simulink model "Aim_23__Monocopter_Testing"  (R2023b)
settings: Solver=ode23t  StartTime=0.0  StopTime=10  MaxStep=1e-3  RelTol=1e-3  AbsTol=1e-3
values from neighbouring files (symbols this model uses):
  air_rho = 1.225    [Aim_23_inherited_params.mat]
  battery_capacity = 22.8    [Aim_23_inherited_params.mat]
  CDO = 10.25    [Aim_23_inherited_params.mat]
  drag_linear = 0.002    [Aim_23_inherited_params.mat]
  drag_quad = 0.005    [Aim_23_inherited_params.mat]
  filtD_motor = 100    [Aim_23_inherited_params.mat]
  filtSpd_motor = 0.001    [Aim_23_inherited_params.mat]
  flap_radius = 0.05312    [Aim_23_inherited_params.mat]
  flap_surface_area = 0.025    [Aim_23_inherited_params.mat]
  kd_motor = 0    [Aim_23_inherited_params.mat]
  ki_motor = 0.00045    [Aim_23_inherited_params.mat]
  klinear = 0.03    [Aim_23_inherited_params.mat]
  kquad = 0.025    [Aim_23_inherited_params.mat]
  limit_motor = 0.25    [Aim_23_inherited_params.mat]
  monoco_mass = 160    [Aim_23_inherited_params.mat]
  monoco_prop =     [Aim_23_inherited_params.mat]
  monoco_radius = 0.61    [Aim_23_inherited_params.mat]
  monoco_wing =     [Aim_23_inherited_params.mat]
  monoco_wing_area = 0.239    [Aim_23_inherited_params.mat]
  waypoints = [-2 -2 0.14 -2 -2 6 0 0 6 2 0 6 ... (15 elements, 3x5)]    [Aim_23_inherited_params.mat]
undefined symbols (not defined in the file or in its folder): X, Y, Z
libraries: sm_lib x97, nesl_utility x38, slpidlib x18, fl_lib x12, sdl_lib x3, simulink x2, simulink_extras x1, batteryecm_lib x1, ee_lib x1
(part 5 of 7)

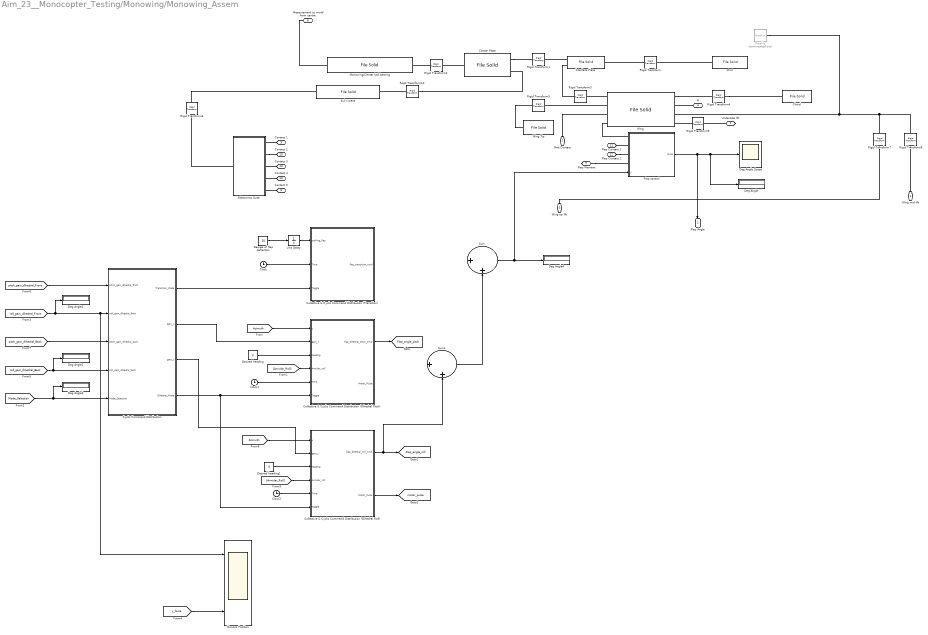
== system Aim_23__Monocopter_Testing/Monowing/Monowing_Assem ==
  " strut" : sm_lib/Body Elements/File Solid  ExtGeomFileName=C:\Users\emman\Monocopter_Frame\DmMc_3mmCF_Strut.STEP  UnitType=FromFile  ExtGeomFileUnits=m  StepReaderType=HEX  ExportConvexHullGeometry=off  InertiaType=CalculateFromGeometry  Mass=5.63  MassUnits=g  CenterOfMass=[0 0 0]  CenterOfMassUnits=m  MomentsOfInertia=[1 1 1]  MomentsOfInertiaUnits=kg*m^2  ProductsOfInertia=[0 0 0]  ProductsOfInertiaUnits=kg*m^2  BasedOnType=Mass  Density=1000  DensityUnits=kg/m^3  DoExposeReferenceFrame=off  SerializedFrames=<Frames><Frame><Id>Frame1</Id><Value><Name>interface</Name><Origin><Source>GeometricFeature</Source><FeatureName>planar surface 6</FeatureName></Origin><PrimaryAxis><DefinedDirection>+Z</DefinedDirection><Source>ReferenceFrame</Source><SourceDirection>+Z</SourceDirection><FeatureName></FeatureName></PrimaryAxis><SecondaryAxis><DefinedDirection>+X</DefinedDirection><Source>ReferenceFrame</Source><SourceDirection>+X</SourceDirection><FeatureName></FeatureName></SecondaryAxis></Value></Frame></Frames>  GraphicType=FromGeometry  MarkerShape=Sphere  MarkerSize=10  GraphicVisPropType=SimpleVisualProperties  GraphicDiffuseColor=[0.5 0.5 0.5]  GraphicSpecularColor=[0.5 0.5 0.5 1.0]  GraphicAmbientColor=[0.15 0.15 0.15 1.0]  GraphicEmissiveColor=[0.0 0.0 0.0 1.0]  GraphicShininess=75  GraphicOpacity=1.0
  Center Plate : sm_lib/Body Elements/File Solid  ExtGeomFileName=C:\Users\emman\Monocopter_Frame\DmMc_center_plate.STEP  UnitType=FromFile  ExtGeomFileUnits=m  StepReaderType=HEX  ExportConvexHullGeometry=off  InertiaType=CalculateFromGeometry  Mass=16.60  MassUnits=g  CenterOfMass=[0 0 0]  CenterOfMassUnits=m  MomentsOfInertia=[1 1 1]  MomentsOfInertiaUnits=kg*m^2  ProductsOfInertia=[0 0 0]  ProductsOfInertiaUnits=kg*m^2  BasedOnType=Mass  Density=1000  DensityUnits=kg/m^3  DoExposeReferenceFrame=on  SerializedFrames=<Frames><Frame><Id>Frame2</Id><Value><Name>interface</Name><Origin><Source>CenterOfMassFrame</Source><FeatureName></FeatureName></Origin><PrimaryAxis><DefinedDirection>+Z</DefinedDirection><Source>ReferenceFrame</Source><SourceDirection>+Z</SourceDirection><FeatureName></FeatureName></PrimaryAxis><SecondaryAxis><DefinedDirection>+X</DefinedDirection><Source>ReferenceFrame</Source><SourceDirection>+X</SourceDirection><FeatureName></FeatureName></SecondaryAxis></Value></Frame><Frame><Id>Frame3</Id><Value><Name>kukri</Name><Origin><Source>CenterOfMassFrame</Source><FeatureName></FeatureName></Origin><PrimaryAxis><DefinedDirection>+Z</DefinedDirection><Source>ReferenceFrame</Source><SourceDirection>+Z</SourceDirection><FeatureName></FeatureName></PrimaryAxis><SecondaryAxis><DefinedDirection>+X</DefinedDirection><Source>ReferenceFrame</Source><SourceDirection>+X</SourceDirection><FeatureName></FeatureName></SecondaryAxis></Value></Frame></Frames>  GraphicType=FromGeometry  MarkerShape=Sphere  MarkerSize=10  GraphicVisPropType=SimpleVisualProperties  GraphicDiffuseColor=[0.5 0.5 0.5]  GraphicSpecularColor=[0.5 0.5 0.5 1.0]  GraphicAmbientColor=[0.15 0.15 0.15 1.0]  GraphicEmissiveColor=[0.0 0.0 0.0 1.0]  GraphicShininess=75  GraphicOpacity=1.0
  Chord : sm_lib/Body Elements/File Solid  ExtGeomFileName=C:\Users\emman\Monocopter_Frame\servo_kukri.STEP  UnitType=FromFile  ExtGeomFileUnits=m  StepReaderType=HEX  ExportConvexHullGeometry=off  InertiaType=CalculateFromGeometry  Mass=8.42  MassUnits=g  CenterOfMass=[0 0 0]  CenterOfMassUnits=m  MomentsOfInertia=[1 1 1]  MomentsOfInertiaUnits=kg*m^2  ProductsOfInertia=[0 0 0]  ProductsOfInertiaUnits=kg*m^2  BasedOnType=Mass  Density=1000  DensityUnits=kg/m^3  DoExposeReferenceFrame=off  SerializedFrames=<Frames><Frame><Id>Frame1</Id><Value><Name>wing</Name><Origin><Source>GeometricFeature</Source><FeatureName>cylindrical surface 54</FeatureName></Origin><PrimaryAxis><DefinedDirection>+Z</DefinedDirection><Source>ReferenceFrame</Source><SourceDirection>+Z</SourceDirection><FeatureName></FeatureName></PrimaryAxis><SecondaryAxis><DefinedDirection>+X</DefinedDirection><Source>ReferenceFrame</Source><SourceDirection>+X</SourceDirection><FeatureName></FeatureName></SecondaryAxis></Value></Frame></Frames>  GraphicType=FromGeometry  MarkerShape=Sphere  MarkerSize=10  GraphicVisPropType=SimpleVisualProperties  GraphicDiffuseColor=[0.5 0.5 0.5]  GraphicSpecularColor=[0.5 0.5 0.5 1.0]  GraphicAmbientColor=[0.15 0.15 0.15 1.0]  GraphicEmissiveColor=[0.0 0.0 0.0 1.0]  GraphicShininess=75  GraphicOpacity=1.0
  Clock : Clock
  Clock1 : Clock
  Clock2 : Clock
  Collective & Cyclic Command Distribution (Dihedral Pitch) : MATLAB Function  TreatAsAtomicUnit=on
  Collective & Cyclic Command Distribution (Dihedral Roll) : MATLAB Function  TreatAsAtomicUnit=on
  Collective & Cyclic Command Distribution (Transition) : MATLAB Function  TreatAsAtomicUnit=on
  Cyclic Command Distribution : MATLAB Function  TreatAsAtomicUnit=on
  Deg Angle{,1..4} (5 alike) : Display
  Deg Angle Scope : Scope
  Degree of flap deflection : Constant  Value=20
  Desired heading : Constant  Value=0
  Desired heading1 : Constant  Value=0
  Electronics Suite : Subsystem
  Flap control : Subsystem
      settings: PortSchema="{\"entries\":[{\"content\":{\"sides\":[{\"content\":{\"connectorIds\":[\"LConn1\",\"LConn2\",\"LConn3\",\"LConn4\",\"In1\"]},\"type\":\"ConnectorPlacement.EquallySpacedRectSide\",\"uuid\":\"1c7c147e-07d6-4292-8f44-26cc109a5078\"},{\"content\":{\"connectorIds\":[\"Out1\"],\"side\":\"RIGHT\"},\"type\":\"ConnectorPlacement.EquallySpacedRectSide\",\"uuid\":\"69a37138-836f-4c0d-80a7-fdf15f5e4c6b\"},{\"content\":{\"connectorIds\":[],\"side\":\"TOP\"},\"type\":\"ConnectorPlacement.EquallySpacedRectSide\",\"uuid\":\"e764985a-8534-4fec-879a-c3123f61d064\"}]},\"type\":\"ConnectorPlacement.EquallySpacedConnector\",\"uuid\":\"d5bc741b-53d2-45d8-8f6d-90823476833a\"}],\"packageUris\":[\"http://schema.mathworks.com/mf0/Connector/R2020b\"],\"version\":\"1.0\"}"
  Graphic : sm_lib/Body Elements/Graphic  Commented=on  GraphicType=Marker  MarkerShape=Cube  MarkerSize=10  GraphicVisPropType=AdvancedVisualProperties  GraphicDiffuseColor=[0.5 0.5 0.5]  GraphicSpecularColor=[0.5 0.5 0.5 1.0]  GraphicAmbientColor=[0.15 0.15 0.15 1.0]  GraphicEmissiveColor=[0.0 0.0 0.0 1.0]  GraphicShininess=75  GraphicOpacity=1.0
  Interface Plate : sm_lib/Body Elements/File Solid  ExtGeomFileName=C:\Users\emman\Monocopter_Frame\new_mid.STEP  UnitType=FromFile  ExtGeomFileUnits=m  StepReaderType=HEX  ExportConvexHullGeometry=off  InertiaType=CalculateFromGeometry  Mass=9.07  MassUnits=g  CenterOfMass=[0 0 0]  CenterOfMassUnits=m  MomentsOfInertia=[1 1 1]  MomentsOfInertiaUnits=kg*m^2  ProductsOfInertia=[0 0 0]  ProductsOfInertiaUnits=kg*m^2  BasedOnType=Mass  Density=1000  DensityUnits=kg/m^3  DoExposeReferenceFrame=off  SerializedFrames=<Frames><Frame><Id>Frame1</Id><Value><Name>interface</Name><Origin><Source>CenterOfMassFrame</Source><FeatureName></FeatureName></Origin><PrimaryAxis><DefinedDirection>+Z</DefinedDirection><Source>ReferenceFrame</Source><SourceDirection>+Z</SourceDirection><FeatureName></FeatureName></PrimaryAxis><SecondaryAxis><DefinedDirection>+X</DefinedDirection><Source>ReferenceFrame</Source><SourceDirection>+X</SourceDirection><FeatureName></FeatureName></SecondaryAxis></Value></Frame><Frame><Id>Frame2</Id><Value><Name>strut</Name><Origin><Source>GeometricFeature</Source><FeatureName>planar surface 30</FeatureName></Origin><PrimaryAxis><DefinedDirection>+Z</DefinedDirection><Source>ReferenceFrame</Source><SourceDirection>+Z</SourceDirection><FeatureName></FeatureName></PrimaryAxis><SecondaryAxis><DefinedDirection>+X</DefinedDirection><Source>ReferenceFrame</Source><SourceDirection>+X</SourceDirection><FeatureName></FeatureName></SecondaryAxis></Value></Frame><Frame><Id>Frame3</Id><Value><Name>wing</Name><Origin><Source>GeometricFeature</Source><FeatureName>planar surface 23</FeatureName></Origin><PrimaryAxis><DefinedDirection>+Z</DefinedDirection><Source>ReferenceFrame</Source><SourceDirection>+Z</SourceDirection><FeatureName></FeatureName></PrimaryAxis><SecondaryAxis><DefinedDirection>+X</DefinedDirection><Source>ReferenceFrame</Source><SourceDirection>+X</SourceDirection><FeatureName></FeatureName></SecondaryAxis></Value></Frame></Frames>  GraphicType=FromGeometry  MarkerShape=Sphere  MarkerSize=10  GraphicVisPropType=SimpleVisualProperties  GraphicDiffuseColor=[0.5 0.5 0.5]  GraphicSpecularColor=[0.5 0.5 0.5 1.0]  GraphicAmbientColor=[0.15 0.15 0.15 1.0]  GraphicEmissiveColor=[0.0 0.0 0.0 1.0]  GraphicShininess=75  GraphicOpacity=1.0
  Kukri piece : sm_lib/Body Elements/File Solid  ExtGeomFileName=C:\Users\emman\Monocopter_Frame\kukri_mid.STEP  UnitType=FromFile  ExtGeomFileUnits=m  StepReaderType=HEX  ExportConvexHullGeometry=off  InertiaType=CalculateFromGeometry  Mass=17.68  MassUnits=g  CenterOfMass=[0 0 0]  CenterOfMassUnits=m  MomentsOfInertia=[1 1 1]  MomentsOfInertiaUnits=kg*m^2  ProductsOfInertia=[0 0 0]  ProductsOfInertiaUnits=kg*m^2  BasedOnType=Mass  Density=1000  DensityUnits=kg/m^3  DoExposeReferenceFrame=off  SerializedFrames=<Frames><Frame><Id>Frame1</Id><Value><Name>Electronics</Name><Origin><Source>GeometricFeature</Source><FeatureName>planar surface 7</FeatureName></Origin><PrimaryAxis><DefinedDirection>+Z</DefinedDirection><Source>ReferenceFrame</Source><SourceDirection>+Z</SourceDirection><FeatureName></FeatureName></PrimaryAxis><SecondaryAxis><DefinedDirection>+X</DefinedDirection><Source>ReferenceFrame</Source><SourceDirection>+X</SourceDirection><FeatureName></FeatureName></SecondaryAxis></Value></Frame><Frame><Id>Frame2</Id><Value><Name>Center_plate</Name><Origin><Source>GeometricFeature</Source><FeatureName>planar surface 11</FeatureName></Origin><PrimaryAxis><DefinedDirection>+Z</DefinedDirection><Source>ReferenceFrame</Source><SourceDirection>+Z</SourceDirection><FeatureName></FeatureName></PrimaryAxis><SecondaryAxis><DefinedDirection>+X</DefinedDirection><Source>ReferenceFrame</Source><SourceDirection>+X</SourceDirection><FeatureName></FeatureName></SecondaryAxis></Value></Frame></Frames>  GraphicType=FromGeometry  MarkerShape=Sphere  MarkerSize=10  GraphicVisPropType=SimpleVisualProperties  GraphicDiffuseColor=[0.5 0.5 0.5]  GraphicSpecularColor=[0.5 0.5 0.5 1.0]  GraphicAmbientColor=[0.15 0.15 0.15 1.0]  GraphicEmissiveColor=[0.0 0.0 0.0 1.0]  GraphicShininess=75  GraphicOpacity=1.0
  Monoco Position : Scope  NumInputPorts=3
  Monowing/Center ball bearing : sm_lib/Body Elements/File Solid  ExtGeomFileName=C:\Users\emman\Monocopter_Frame\DmMc_Ball_Bearing.STEP  UnitType=FromFile  ExtGeomFileUnits=m  StepReaderType=HEX  ExportConvexHullGeometry=off  InertiaType=CalculateFromGeometry  Mass=3.04  MassUnits=g  CenterOfMass=[0 0 0]  CenterOfMassUnits=m  MomentsOfInertia=[0.0001 0.001 0.001]  MomentsOfInertiaUnits=kg*m^2  ProductsOfInertia=[0 0 0]  ProductsOfInertiaUnits=kg*m^2  BasedOnType=Mass  Density=1000  DensityUnits=kg/m^3  DoExposeReferenceFrame=on  SerializedFrames=<Frames><Frame><Id>Frame1</Id><Value><Name>Measurement to world</Name><Origin><Source>ReferenceFrame</Source><FeatureName></FeatureName></Origin><PrimaryAxis><DefinedDirection>+Z</DefinedDirection><Source>ReferenceFrame</Source><SourceDirection>+Z</SourceDirection><FeatureName></FeatureName></PrimaryAxis><SecondaryAxis><DefinedDirection>+X</DefinedDirection><Source>ReferenceFrame</Source><SourceDirection>+X</SourceDirection><FeatureName></FeatureName></SecondaryAxis></Value></Frame></Frames>  GraphicType=FromGeometry  MarkerShape=Sphere  MarkerSize=10  GraphicVisPropType=SimpleVisualProperties  GraphicDiffuseColor=[0.2 0.2 0.2]  GraphicSpecularColor=[0.5 0.5 0.5 1.0]  GraphicAmbientColor=[0.15 0.15 0.15 1.0]  GraphicEmissiveColor=[0.0 0.0 0.0 1.0]  GraphicShininess=75  GraphicOpacity=1.0
  Rigid Transform : sm_lib/Frames and Transforms/Rigid Transform  TranslationMethod=Cartesian  TranslationStandardOffset=0  TranslationStandardOffsetUnits=mm  TranslationStandardAxis=+Z  TranslationCartesianOffset=[0 0 0]  TranslationCartesianOffsetUnits=mm  TranslationROffset=0  TranslationROffsetUnits=m  TranslationZOffset=0  TranslationZOffsetUnits=m  TranslationThetaOffset=0  TranslationThetaOffsetUnits=deg  RotationMethod=RotationSequence  RotationAngleUnits=deg  RotationStandardAxis=+Z  RotationAngle=0.0  RotationArbitraryAxis=[0 0 1]  FollAlignAxisA=+X  BaseAlignAxisA=+Y  FollAlignAxisB=+Y  BaseAlignAxisB=+Z  RotationSequenceAxes=FollowerAxes  RotationSequence=YZX  RotationSequenceAngles=[180 1 -11]  RotationSequenceAnglesUnits=deg  RotationMatrix=[1 0 0; 0 1 0; 0 0 1]  Quaternion=[1 0 0 0]
  Rigid Transform1 : sm_lib/Frames and Transforms/Rigid Transform  TranslationMethod=Cartesian  TranslationStandardOffset=0  TranslationStandardOffsetUnits=mm  TranslationStandardAxis=+Z  TranslationCartesianOffset=[47 -2.5 1.2]  TranslationCartesianOffsetUnits=mm  TranslationROffset=0  TranslationROffsetUnits=m  TranslationZOffset=0  TranslationZOffsetUnits=m  TranslationThetaOffset=0  TranslationThetaOffsetUnits=deg  RotationMethod=RotationSequence  RotationAngleUnits=deg  RotationStandardAxis=+Z  RotationAngle=0.0  RotationArbitraryAxis=[0 0 1]  FollAlignAxisA=+X  BaseAlignAxisA=+Y  FollAlignAxisB=+Y  BaseAlignAxisB=+Z  RotationSequenceAxes=FollowerAxes  RotationSequence=ZXZ  RotationSequenceAngles=[180 0 0]  RotationSequenceAnglesUnits=deg  RotationMatrix=[1 0 0; 0 1 0; 0 0 1]  Quaternion=[1 0 0 0]
  Rigid Transform10 : sm_lib/Frames and Transforms/Rigid Transform  TranslationMethod=Cartesian  TranslationStandardOffset=0  TranslationStandardOffsetUnits=mm  TranslationStandardAxis=+Z  TranslationCartesianOffset=[-27.5 0 0]  TranslationCartesianOffsetUnits=mm  TranslationROffset=0  TranslationROffsetUnits=m  TranslationZOffset=0  TranslationZOffsetUnits=m  TranslationThetaOffset=0  TranslationThetaOffsetUnits=deg  RotationMethod=None  RotationAngleUnits=deg  RotationStandardAxis=+Z  RotationAngle=0.0  RotationArbitraryAxis=[0 0 1]  FollAlignAxisA=+X  BaseAlignAxisA=+Y  FollAlignAxisB=+Y  BaseAlignAxisB=+Z  RotationSequenceAxes=FollowerAxes  RotationSequence=XYX  RotationSequenceAngles=[0 0 0]  RotationSequenceAnglesUnits=deg  RotationMatrix=[1 0 0; 0 1 0; 0 0 1]  Quaternion=[1 0 0 0]
  Rigid Transform2 : sm_lib/Frames and Transforms/Rigid Transform  TranslationMethod=Cartesian  TranslationStandardOffset=0  TranslationStandardOffsetUnits=mm  TranslationStandardAxis=+Z  TranslationCartesianOffset=[0 0 -4]  TranslationCartesianOffsetUnits=mm  TranslationROffset=0  TranslationROffsetUnits=m  TranslationZOffset=0  TranslationZOffsetUnits=m  TranslationThetaOffset=0  TranslationThetaOffsetUnits=deg  RotationMethod=None  RotationAngleUnits=deg  RotationStandardAxis=+Z  RotationAngle=0.0  RotationArbitraryAxis=[0 0 1]  FollAlignAxisA=+X  BaseAlignAxisA=+Y  FollAlignAxisB=+Y  BaseAlignAxisB=+Z  RotationSequenceAxes=FollowerAxes  RotationSequence=XYX  RotationSequenceAngles=[0 0 0]  RotationSequenceAnglesUnits=deg  RotationMatrix=[1 0 0; 0 1 0; 0 0 1]  Quaternion=[1 0 0 0]
  Rigid Transform3 : sm_lib/Frames and Transforms/Rigid Transform  TranslationMethod=Cartesian  TranslationStandardOffset=0  TranslationStandardOffsetUnits=mm  TranslationStandardAxis=+Z  TranslationCartesianOffset=[-186.3 -36.8 7.7]  TranslationCartesianOffsetUnits=mm  TranslationROffset=0  TranslationROffsetUnits=m  TranslationZOffset=0  TranslationZOffsetUnits=m  TranslationThetaOffset=0  TranslationThetaOffsetUnits=deg  RotationMethod=RotationSequence  RotationAngleUnits=deg  RotationStandardAxis=+Z  RotationAngle=0.0  RotationArbitraryAxis=[0 0 1]  FollAlignAxisA=+X  BaseAlignAxisA=+Y  FollAlignAxisB=+Y  BaseAlignAxisB=+Z  RotationSequenceAxes=FollowerAxes  RotationSequence=XYX  RotationSequenceAngles=[-12 0 0]  RotationSequenceAnglesUnits=deg  RotationMatrix=[1 0 0; 0 1 0; 0 0 1]  Quaternion=[1 0 0 0]
  Rigid Transform4 : sm_lib/Frames and Transforms/Rigid Transform  TranslationMethod=Cartesian  TranslationStandardOffset=0  TranslationStandardOffsetUnits=mm  TranslationStandardAxis=+Z  TranslationCartesianOffset=[0.4 5 0.6]  TranslationCartesianOffsetUnits=mm  TranslationROffset=0  TranslationROffsetUnits=m  TranslationZOffset=0  TranslationZOffsetUnits=m  TranslationThetaOffset=0  TranslationThetaOffsetUnits=deg  RotationMethod=RotationSequence  RotationAngleUnits=deg  RotationStandardAxis=+Z  RotationAngle=0.0  RotationArbitraryAxis=[0 0 1]  FollAlignAxisA=+X  BaseAlignAxisA=+Y  FollAlignAxisB=+Y  BaseAlignAxisB=+Z  RotationSequenceAxes=FollowerAxes  RotationSequence=XYX  RotationSequenceAngles=[10 2 0]  RotationSequenceAnglesUnits=deg  RotationMatrix=[1 0 0; 0 1 0; 0 0 1]  Quaternion=[1 0 0 0]
  Rigid Transform5 : sm_lib/Frames and Transforms/Rigid Transform  TranslationMethod=Cartesian  TranslationStandardOffset=0  TranslationStandardOffsetUnits=mm  TranslationStandardAxis=+Z  TranslationCartesianOffset=[6 14.65 3.1]  TranslationCartesianOffsetUnits=mm  TranslationROffset=0  TranslationROffsetUnits=m  TranslationZOffset=0  TranslationZOffsetUnits=m  TranslationThetaOffset=0  TranslationThetaOffsetUnits=deg  RotationMethod=RotationSequence  RotationAngleUnits=deg  RotationStandardAxis=+Z  RotationAngle=0.0  RotationArbitraryAxis=[0 0 1]  FollAlignAxisA=+X  BaseAlignAxisA=+Y  FollAlignAxisB=+Y  BaseAlignAxisB=+Z  RotationSequenceAxes=FollowerAxes  RotationSequence=XYX  RotationSequenceAngles=[12 2 0]  RotationSequenceAnglesUnits=deg  RotationMatrix=[1 0 0; 0 1 0; 0 0 1]  Quaternion=[1 0 0 0]
  Rigid Transform6 : sm_lib/Frames and Transforms/Rigid Transform  TranslationMethod=Cartesian  TranslationStandardOffset=0  TranslationStandardOffsetUnits=mm  TranslationStandardAxis=+Z  TranslationCartesianOffset=[-72.7 -18.05 2.83]  TranslationCartesianOffsetUnits=mm  TranslationROffset=0  TranslationROffsetUnits=m  TranslationZOffset=0  TranslationZOffsetUnits=m  TranslationThetaOffset=0  TranslationThetaOffsetUnits=deg  RotationMethod=RotationSequence  RotationAngleUnits=deg  RotationStandardAxis=+Z  RotationAngle=0.0  RotationArbitraryAxis=[0 0 1]  FollAlignAxisA=+X  BaseAlignAxisA=+Y  FollAlignAxisB=+Y  BaseAlignAxisB=+Z  RotationSequenceAxes=FollowerAxes  RotationSequence=XYZ  RotationSequenceAngles=[180 180.4 15.0]  RotationSequenceAnglesUnits=deg  RotationMatrix=[1 0 0; 0 1 0; 0 0 1]  Quaternion=[1 0 0 0]
  Rigid Transform7 : sm_lib/Frames and Transforms/Rigid Transform  TranslationMethod=Cartesian  TranslationStandardOffset=0  TranslationStandardOffsetUnits=mm  TranslationStandardAxis=+Z  TranslationCartesianOffset=[0 55 80]  TranslationCartesianOffsetUnits=mm  TranslationROffset=0  TranslationROffsetUnits=m  TranslationZOffset=0  TranslationZOffsetUnits=m  TranslationThetaOffset=0  TranslationThetaOffsetUnits=deg  RotationMethod=RotationSequence  RotationAngleUnits=deg  RotationStandardAxis=+Z  RotationAngle=0.0  RotationArbitraryAxis=[0 0 1]  FollAlignAxisA=+X  BaseAlignAxisA=+Y  FollAlignAxisB=+Y  BaseAlignAxisB=+Z  RotationSequenceAxes=FollowerAxes  RotationSequence=XYZ  RotationSequenceAngles=[10 0 0]  RotationSequenceAnglesUnits=deg  RotationMatrix=[1 0 0; 0 1 0; 0 0 1]  Quaternion=[1 0 0 0]
  Rigid Transform8 : sm_lib/Frames and Transforms/Rigid Transform  TranslationMethod=Cartesian  TranslationStandardOffset=0  TranslationStandardOffsetUnits=mm  TranslationStandardAxis=+Z  TranslationCartesianOffset=[0 60 15]  TranslationCartesianOffsetUnits=mm  TranslationROffset=0  TranslationROffsetUnits=m  TranslationZOffset=0  TranslationZOffsetUnits=m  TranslationThetaOffset=0  TranslationThetaOffsetUnits=deg  RotationMethod=None  RotationAngleUnits=deg  RotationStandardAxis=+Z  RotationAngle=0.0  RotationArbitraryAxis=[0 0 1]  FollAlignAxisA=+X  BaseAlignAxisA=+Y  FollAlignAxisB=+Y  BaseAlignAxisB=+Z  RotationSequenceAxes=FollowerAxes  RotationSequence=XYX  RotationSequenceAngles=[0 0 0]  RotationSequenceAnglesUnits=deg  RotationMatrix=[1 0 0; 0 1 0; 0 0 1]  Quaternion=[1 0 0 0]
  Rigid Transform9 : sm_lib/Frames and Transforms/Rigid Transform  TranslationMethod=None  TranslationStandardOffset=0  TranslationStandardOffsetUnits=m  TranslationStandardAxis=+Z  TranslationCartesianOffset=[0 0 0]  TranslationCartesianOffsetUnits=m  TranslationROffset=0  TranslationROffsetUnits=m  TranslationZOffset=0  TranslationZOffsetUnits=m  TranslationThetaOffset=0  TranslationThetaOffsetUnits=deg  RotationMethod=None  RotationAngleUnits=deg  RotationStandardAxis=+Z  RotationAngle=0.0  RotationArbitraryAxis=[0 0 1]  FollAlignAxisA=+X  BaseAlignAxisA=+Y  FollAlignAxisB=+Y  BaseAlignAxisB=+Z  RotationSequenceAxes=FollowerAxes  RotationSequence=XYX  RotationSequenceAngles=[0 0 0]  RotationSequenceAnglesUnits=deg  RotationMatrix=[1 0 0; 0 1 0; 0 0 1]  Quaternion=[1 0 0 0]
  Sum : Sum  Inputs=|++
  Sum1 : Sum  Inputs=|++
  Unit Delay : UnitDelay  SampleTime=7.2  HasFrameUpgradeWarning=on
  Wing : sm_lib/Body Elements/File Solid  ExtGeomFileName=C:\Users\emman\Monocopter_Frame\DmMc_Wing_type7_Flap.STEP  UnitType=FromFile  ExtGeomFileUnits=m  StepReaderType=HEX  ExportConvexHullGeometry=off  InertiaType=CalculateFromGeometry  Mass=1.98  MassUnits=g  CenterOfMass=[0 0 0]  CenterOfMassUnits=m  MomentsOfInertia=[1 1 1]  MomentsOfInertiaUnits=kg*m^2  ProductsOfInertia=[0 0 0]  ProductsOfInertiaUnits=kg*m^2  BasedOnType=Mass  Density=0.016  DensityUnits=g/cm^3  DoExposeReferenceFrame=off  SerializedFrames=<Frames><Frame><Id>Frame1</Id><Value><Name>interface</Name><Origin><Source>CenterOfMassFrame</Source><FeatureName></FeatureName></Origin><PrimaryAxis><DefinedDirection>+Z</DefinedDirection><Source>ReferenceFrame</Source><SourceDirection>+Z</SourceDirection><FeatureName></FeatureName></PrimaryAxis><SecondaryAxis><DefinedDirection>+X</DefinedDirection><Source>ReferenceFrame</Source><SourceDirection>+X</SourceDirection><FeatureName></FeatureName></SecondaryAxis></Value></Frame><Frame><Id>Frame2</Id><Value><Name>chord</Name><Origin><Source>GeometricFeature</Source><FeatureName>planar surface 25</FeatureName></Origin><PrimaryAxis><DefinedDirection>+Z</DefinedDirection><Source>ReferenceFrame</Source><SourceDirection>+Z</SourceDirection><FeatureName></FeatureName></PrimaryAxis><SecondaryAxis><DefinedDirection>+X</DefinedDirection><Source>ReferenceFrame</Source><SourceDirection>+X</SourceDirection><FeatureName></FeatureName></SecondaryAxis></Value></Frame><Frame><Id>Frame3</Id><Value><Name>Wing Tip</Name><Origin><Source>GeometricFeature</Source><FeatureName>general surface 1</FeatureName></Origin><PrimaryAxis><DefinedDirection>+Z</DefinedDirection><Source>ReferenceFrame</Source><SourceDirection>+Z</SourceDirection><FeatureName></FeatureName></PrimaryAxis><SecondaryAxis><DefinedDirection>+X</DefinedDirection><Source>ReferenceFrame</Source><SourceDirection>+X</SourceDirection><FeatureName></FeatureName></SecondaryAxis></Value></Frame><Frame><Id>Frame4</Id><Value><Name>Mount</Name><Origin><Source>ReferenceFrame</Source><FeatureName></FeatureName></Origin><PrimaryAxis><DefinedDirection>+Z</DefinedDirection><Source>ReferenceFrame</Source><SourceDirection>+Z</SourceDirection><FeatureName></FeatureName></PrimaryAxis><SecondaryAxis><DefinedDirection>+X</DefinedDirection><Source>ReferenceFrame</Source><SourceDirection>+X</SourceDirection><FeatureName></FeatureName></SecondaryAxis></Value></Frame><Frame><Id>Frame5</Id><Value><Name>Gnd_Contact</Name><Origin><Source>GeometricFeature</Source><FeatureName>segment 50</FeatureName></Origin><PrimaryAxis><DefinedDirection>+Z</DefinedDirection><Source>ReferenceFrame</Source><SourceDirection>+Z</SourceDirection><FeatureName></FeatureName></PrimaryAxis><SecondaryAxis><DefinedDirection>+X</DefinedDirection><Source>ReferenceFrame</Source><SourceDirection>+X</SourceDirection><FeatureName></FeatureName></SecondaryAxis></Value></Frame><Frame><Id>Frame6</Id><Value><Name>Lift</Name><Origin><Source>CenterOfMassFrame</Source><FeatureName></FeatureName></Origin><PrimaryAxis><DefinedDirection>+Z</DefinedDirection><Source>ReferenceFrame</Source><SourceDirection>+Z</SourceDirection><FeatureName></FeatureName></PrimaryAxis><SecondaryAxis><DefinedDirection>+X</DefinedDirection><Source>ReferenceFrame</Source><SourceDirection>+X</SourceDirection><FeatureName></FeatureName></SecondaryAxis></Value></Frame><Frame><Id>Frame7</Id><Value><Name>Flap</Name><Origin><Source>GeometricFeature</Source><FeatureName>segment 11</FeatureName></Origin><PrimaryAxis><DefinedDirection>+Z</DefinedDirection><Source>GeometricFeature</Source><SourceDirection>+Z</SourceDirection><FeatureName>segment 11</FeatureName></PrimaryAxis><SecondaryAxis><DefinedDirection>+X</DefinedDirection><Source>ReferenceFrame</Source><SourceDirection>+X</SourceDirection><FeatureName></FeatureName></SecondaryAxis></Value></Frame><Frame><Id>Frame8</Id><Value><Name>Lift_underside</Name><Origin><Source>CenterOfMassFrame</Source><FeatureName></FeatureName></Origin><PrimaryAxis><DefinedDirection>-Z</DefinedDirection><Source>ReferenceFrame</Source><SourceDirection>+Z</SourceDirection><FeatureName></FeatureName></PrimaryAxis><SecondaryAxis><DefinedDirection>+X</DefinedDirection><Source>ReferenceFrame</Source><SourceDirection>+X</SourceDirection><FeatureName></FeatureName></SecondaryAxis></Value></Frame></Frames>  GraphicType=FromGeometry  MarkerShape=Sphere  MarkerSize=10  GraphicVisPropType=SimpleVisualProperties  GraphicDiffuseColor=[1.0 1.0 0.2]  GraphicSpecularColor=[0.5 0.5 0.5 1.0]  GraphicAmbientColor=[0.15 0.15 0.15 1.0]  GraphicEmissiveColor=[0.0 0.0 0.0 1.0]  GraphicShininess=75  GraphicOpacity=1.0
  Wing Tip : sm_lib/Body Elements/File Solid  ExtGeomFileName=C:\Users\emman\Monocopter_Frame\DmMc_Wingtip_Rinforce_type6.STEP  UnitType=FromFile  ExtGeomFileUnits=m  StepReaderType=HEX  ExportConvexHullGeometry=off  InertiaType=CalculateFromGeometry  Mass=2.5  MassUnits=g  CenterOfMass=[0 0 0]  CenterOfMassUnits=m  MomentsOfInertia=[1 1 1]  MomentsOfInertiaUnits=kg*m^2  ProductsOfInertia=[0 0 0]  ProductsOfInertiaUnits=kg*m^2  BasedOnType=Mass  Density=1000  DensityUnits=kg/m^3  DoExposeReferenceFrame=off  SerializedFrames=<Frames><Frame><Id>Frame1</Id><Value><Name>Wing</Name><Origin><Source>GeometricFeature</Source><FeatureName>general surface 8</FeatureName></Origin><PrimaryAxis><DefinedDirection>+Z</DefinedDirection><Source>ReferenceFrame</Source><SourceDirection>+Z</SourceDirection><FeatureName></FeatureName></PrimaryAxis><SecondaryAxis><DefinedDirection>+X</DefinedDirection><Source>ReferenceFrame</Source><SourceDirection>+X</SourceDirection><FeatureName></FeatureName></SecondaryAxis></Value></Frame></Frames>  GraphicType=FromGeometry  MarkerShape=Sphere  MarkerSize=10  GraphicVisPropType=SimpleVisualProperties  GraphicDiffuseColor=[0.5 0.5 0.5]  GraphicSpecularColor=[0.5 0.5 0.5 1.0]  GraphicAmbientColor=[0.15 0.15 0.15 1.0]  GraphicEmissiveColor=[0.0 0.0 0.0 1.0]  GraphicShininess=75  GraphicOpacity=1.0
  Wing mid lift : PMIOPort  Side=Left
  Underside lift : PMIOPort  Port=2  Side=Left
  Wing tip lift : PMIOPort  Port=3  Side=Left
  M : PMIOPort  Port=4  Side=Left
  Flap Moment : PMIOPort  Port=5  Side=Left
  Contact 5 : PMIOPort  Port=6  Side=Left
  Gnd Contact : PMIOPort  Port=7  Side=Right
  Measurement to world from centre : PMIOPort  Port=8  Side=Right
  Contact 1 : PMIOPort  Port=9  Side=Right
  Contact 2 : PMIOPort  Port=10  Side=Right
  Flap Contact 1 : PMIOPort  Port=11  Side=Right
  Flap Contact 2 : PMIOPort  Port=12  Side=Right
  Contact 3 : PMIOPort  Port=13  Side=Right
  Contact 4 : PMIOPort  Port=14  Side=Right
  Flap Angle : Outport
  tag scope: Flap_angle_pitch=global, Flap_angle_roll=global, motor_pulse=global
  wires:
  Flap control/1(Out1) -> Flap Angle/1, Deg Angle/1, Deg Angle Scope/1
  Degree of flap deflection/1 -> Unit Delay/1
  Clock/1 -> Collective & Cyclic Command Distribution (Transition)/2(Time)
  Unit Delay/1 -> Collective & Cyclic Command Distribution (Transition)/1(stalling_flap)
  [Annular_Roll] -> Collective & Cyclic Command Distribution (Dihedral Pitch)/4(Annular_roll)
  Desired heading/1 -> Collective & Cyclic Command Distribution (Dihedral Pitch)/3(heading)
  [Azimuth] -> Collective & Cyclic Command Distribution (Dihedral Pitch)/1(u)
  Clock1/1 -> Collective & Cyclic Command Distribution (Dihedral Pitch)/5(Time)
  Cyclic Command Distribution/1(Transition_Mode) -> Collective & Cyclic Command Distribution (Transition)/3(Toggle)
  Cyclic Command Distribution/2(gain_x) -> Collective & Cyclic Command Distribution (Dihedral Pitch)/2(gain_x)
  [Mode_Selection] -> Cyclic Command Distribution/5(Mode_Selection), Deg Angle3/1
  [roll_gain_dihedral_Front] -> Monoco Position/1, Cyclic Command Distribution/2(roll_gain_dihedral_front), Deg Angle1/1
  [roll_gain_dihedral_Back] -> Deg Angle2/1, Cyclic Command Distribution/4(roll_gain_dihedral_back)
  Sum/1 -> Deg Angle4/1, Flap control/1(y)
  Cyclic Command Distribution/4(Dihedral_Mode) -> Collective & Cyclic Command Distribution (Dihedral Roll)/6(Toggle), Collective & Cyclic Command Distribution (Dihedral Pitch)/6(Toggle)
  [y_force] -> Monoco Position/3
  [pitch_gain_dihedral_Front] -> Cyclic Command Distribution/1(pitch_gain_dihedral_front)
  [pitch_gain_dihedral_Back] -> Cyclic Command Distribution/3(pitch_gain_dihedral_back)
  Cyclic Command Distribution/3(gain_y) -> Collective & Cyclic Command Distribution (Dihedral Roll)/2(gain_y)
  [Azimuth] -> Collective & Cyclic Command Distribution (Dihedral Roll)/1(u)
  Desired heading1/1 -> Collective & Cyclic Command Distribution (Dihedral Roll)/3(heading)
  [Annular_Roll] -> Collective & Cyclic Command Distribution (Dihedral Roll)/4(Annular_roll)
  Clock2/1 -> Collective & Cyclic Command Distribution (Dihedral Roll)/5(Time)
  Collective & Cyclic Command Distribution (Dihedral Pitch)/1(flap_dihedral_pitch_cmd) -> [Flap_angle_pitch]
  Collective & Cyclic Command Distribution (Dihedral Roll)/1(flap_dihedral_roll_cmd) -> [Flap_angle_roll], Sum1/2
  Sum1/1 -> Sum/2
  Collective & Cyclic Command Distribution (Dihedral Roll)/2(Motor_Pulse) -> [motor_pulse]
  connections:
  Rigid Transform4/RConn1 -- Chord/LConn1
  Wing/RConn1 -- Rigid Transform4/LConn1
  Rigid Transform/LConn1 -- Interface Plate/RConn1
  Rigid Transform2/LConn1 -- Monowing/Center ball bearing/RConn1
  Interface Plate/LConn1 -- Rigid Transform1/RConn1
  M/RConn1 -- Wing/RConn2
  Wing/LConn1 -- Rigid Transform3/RConn1
  Wing/LConn2 -- Rigid Transform5/LConn1
  Center Plate/RConn1 -- Rigid Transform2/RConn1
  " strut"/LConn1 -- Rigid Transform/RConn1
  Rigid Transform3/LConn1 -- Interface Plate/LConn2
  Rigid Transform5/RConn1 -- Wing Tip/LConn1
  Center Plate/LConn1 -- Rigid Transform1/LConn1
  Wing/LConn3 -- Gnd Contact/RConn1
  Contact 1/RConn1 -- Electronics Suite/RConn1
  Electronics Suite/LConn1 -- Rigid Transform6/RConn1
  Electronics Suite/RConn2 -- Contact 2/RConn1
  Monowing/Center ball bearing/LConn1 -- Measurement to world from centre/RConn1
  Rigid Transform7/RConn1 -- Wing tip lift/RConn1
  Rigid Transform7/LConn1 -- Wing/RConn3 -- Graphic/RConn1 -- Rigid Transform8/LConn1
  Wing mid lift/RConn1 -- Rigid Transform8/RConn1
  Flap control/LConn1 -- Wing/LConn4
  Rigid Transform9/LConn1 -- Wing/RConn4
  Underside lift/RConn1 -- Rigid Transform9/RConn1
  Flap control/LConn2 -- Flap Contact 1/RConn1
  Flap Contact 2/RConn1 -- Flap control/LConn3
  Contact 3/RConn1 -- Electronics Suite/RConn3
  Contact 4/RConn1 -- Electronics Suite/RConn4
  Contact 5/RConn1 -- Electronics Suite/RConn5
  Rigid Transform6/LConn1 -- Kukri piece/LConn1
  Rigid Transform10/RConn1 -- Kukri piece/RConn1
  Rigid Transform10/LConn1 -- Center Plate/LConn2
  Flap Moment/RConn1 -- Flap control/LConn4

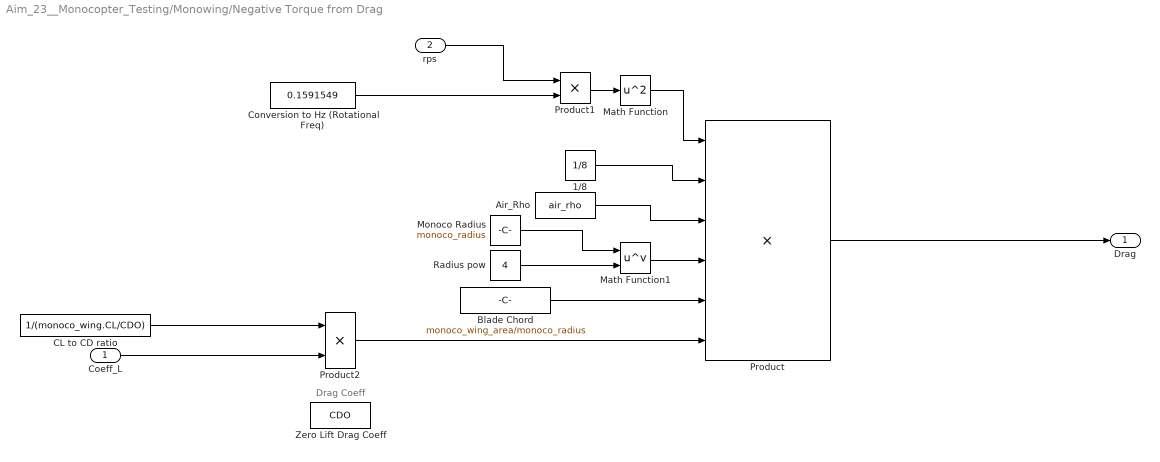
== system Aim_23__Monocopter_Testing/Monowing/Negative Torque from Drag ==
  note: Drag Coeff
  Coeff_L : Inport
  rps : Inport  Port=2
  1/8 : Constant  Value=1/8
  Air_Rho : Constant  Value=air_rho
  Blade Chord : Constant  Value=monoco_wing_area/monoco_radius
  CL to CD ratio : Constant  Value=1/(monoco_wing.CL/CDO)
  Conversion to Hz (Rotational Freq) : Constant  Value=0.1591549
  Math Function : Math  Operator=square
  Math Function1 : Math  Operator=pow
  Monoco Radius : Constant  Value=monoco_radius
  Product : Product  Inputs=6
  Product1 : Product
  Product2 : Product
  Radius pow : Constant  Value=4
  Zero Lift Drag Coeff : Constant  Value=CDO
  Drag : Outport
  wires:
  Math Function1/1 -> Product/4
  Product/1 -> Drag/1
  Conversion to Hz (Rotational Freq)/1 -> Product1/2
  Air_Rho/1 -> Product/3
  Product1/1 -> Math Function/1
  Radius pow/1 -> Math Function1/2
  Math Function/1 -> Product/1
  Blade Chord/1 -> Product/5
  rps/1 -> Product1/1
  Monoco Radius/1 -> Math Function1/1
  1/8/1 -> Product/2
  CL to CD ratio/1 -> Product2/1
  Coeff_L/1 -> Product2/2
  Product2/1 -> Product/6

== system Aim_23__Monocopter_Testing/Monowing/Speed Brake mode ==
  rps : Inport
  Clock1 : Clock
  Pitch : Display
  Speed Brake Mode Activation : MATLAB Function  TreatAsAtomicUnit=on
  Added Drag : Outport
  wires:
  [Body_Pitch] -> Pitch/1, Speed Brake Mode Activation/2(pitch)
  [Mode_Selection] -> Speed Brake Mode Activation/4(Mode)
  rps/1 -> Speed Brake Mode Activation/1(rps)
  Clock1/1 -> Speed Brake Mode Activation/3(Time)
  Speed Brake Mode Activation/1(y) -> Added Drag/1

== system Aim_23__Monocopter_Testing/Collective Control/PD Alt Controller (Monoco negative direction counter clockwise)/Low Pass Filter ==
  In2 : Inport
  If : If  IfExpression=u1<(-2200)
  If Action Subsystem : Subsystem  TreatAsAtomicUnit=on
  If Action Subsystem1 : Subsystem  TreatAsAtomicUnit=on
  Maximum Allowable : Constant  Value=-2200
  Merge : Merge
  u : Outport
  wires:
  Merge/1 -> u/1
  If/2 -> If Action Subsystem/Action
  If Action Subsystem/1(Out1) -> Merge/2
  If Action Subsystem1/1(Out1) -> Merge/1
  In2/1 -> If Action Subsystem/1(In1), If/1
  Maximum Allowable/1 -> If Action Subsystem1/1(In1)
  If/1 -> If Action Subsystem1/Action

== system Aim_23__Monocopter_Testing/Collective Control/PD Alt Controller (Monoco negative direction counter clockwise)/Offset ==
  In2 : Inport
  Offset : Constant  Value=0.2
  Subtract1 : Sum
  Out1 : Outport
  wires:
  In2/1 -> Subtract1/1
  Offset/1 -> Subtract1/2
  Subtract1/1 -> Out1/1

== system Aim_23__Monocopter_Testing/Collective Control/PD Alt Controller (Monoco positve direction clockwise)/Low Pass Filter ==
  In2 : Inport
  If : If  IfExpression=u1>(2300)
  If Action Subsystem : Subsystem  TreatAsAtomicUnit=on
  If Action Subsystem1 : Subsystem  TreatAsAtomicUnit=on
  Maximum Allowable : Constant  Value=2300
  Merge : Merge
  u : Outport
  wires:
  Merge/1 -> u/1
  If/2 -> If Action Subsystem/Action
  If Action Subsystem/1(Out1) -> Merge/2
  If Action Subsystem1/1(Out1) -> Merge/1
  In2/1 -> If Action Subsystem/1(In1), If/1
  Maximum Allowable/1 -> If Action Subsystem1/1(In1)
  If/1 -> If Action Subsystem1/Action

== system Aim_23__Monocopter_Testing/Collective Control/PD Alt Controller (Monoco positve direction clockwise)/Offset ==
  In2 : Inport
  Offset : Constant  Value=0.2
  Subtract1 : Sum
  Out1 : Outport
  wires:
  In2/1 -> Subtract1/1
  Offset/1 -> Subtract1/2
  Subtract1/1 -> Out1/1

== system Aim_23__Monocopter_Testing/Control Modules/Bang Bang Control/If Action Subsystem ==
  In1 : Inport
  Action Port : ActionPort  ActionPortLabel=else
  Out1 : Outport
  wires:
  In1/1 -> Out1/1

== system Aim_23__Monocopter_Testing/Control Modules/Bang Bang Control/If Action Subsystem1 ==
  In1 : Inport
  Action Port : ActionPort  ActionPortLabel=if(u1 > 1)
  Out1 : Outport
  wires:
  In1/1 -> Out1/1

== system Aim_23__Monocopter_Testing/Control Modules/Bang Bang Control Ideal/If Action Subsystem ==
  In1 : Inport
  Action Port : ActionPort  ActionPortLabel=else
  Out1 : Outport
  wires:
  In1/1 -> Out1/1

== system Aim_23__Monocopter_Testing/Control Modules/Bang Bang Control Ideal/If Action Subsystem1 ==
  In1 : Inport
  Action Port : ActionPort  ActionPortLabel=if(u1 > 1)
  Out1 : Outport
  wires:
  In1/1 -> Out1/1

== system Aim_23__Monocopter_Testing/Control Modules/Subsystem/If Action Subsystem ==
  In1 : Inport
  Action Port : ActionPort  ActionPortLabel=else
  Out1 : Outport
  wires:
  In1/1 -> Out1/1

== system Aim_23__Monocopter_Testing/Control Modules/Subsystem/If Action Subsystem1 ==
  In1 : Inport
  Action Port : ActionPort  ActionPortLabel=if(u1<(-40))
  Out1 : Outport
  wires:
  In1/1 -> Out1/1

== system Aim_23__Monocopter_Testing/Cyclic Roll Control/PD Pitch Controller (Monoco negative direction counter clockwise) Back Motor/Low Pass Filter ==
  In2 : Inport
  If : If  IfExpression=u1<(-2300)
  If Action Subsystem : Subsystem  TreatAsAtomicUnit=on
  If Action Subsystem1 : Subsystem  TreatAsAtomicUnit=on
  Maximum Allowable : Constant  Value=-2300
  Merge : Merge
  u : Outport
  wires:
  Merge/1 -> u/1
  If/2 -> If Action Subsystem/Action
  If Action Subsystem/1(Out1) -> Merge/2
  If Action Subsystem1/1(Out1) -> Merge/1
  In2/1 -> If Action Subsystem/1(In1), If/1
  Maximum Allowable/1 -> If Action Subsystem1/1(In1)
  If/1 -> If Action Subsystem1/Action

== system Aim_23__Monocopter_Testing/Cyclic Roll Control/PD Pitch Controller (Monoco negative direction counter clockwise) Back Motor/Offset ==
  In2 : Inport
  Offset : Constant  Value=0.2
  Subtract1 : Sum
  Out1 : Outport
  wires:
  In2/1 -> Subtract1/1
  Offset/1 -> Subtract1/2
  Subtract1/1 -> Out1/1

== system Aim_23__Monocopter_Testing/Cyclic Roll Control/PD Pitch Controller (Monoco negative direction counter clockwise) Front Motor/Low Pass Filter ==
  In2 : Inport
  If : If  IfExpression=u1<(-2300)
  If Action Subsystem : Subsystem  TreatAsAtomicUnit=on
  If Action Subsystem1 : Subsystem  TreatAsAtomicUnit=on
  Maximum Allowable : Constant  Value=-2300
  Merge : Merge
  u : Outport
  wires:
  Merge/1 -> u/1
  If/2 -> If Action Subsystem/Action
  If Action Subsystem/1(Out1) -> Merge/2
  If Action Subsystem1/1(Out1) -> Merge/1
  In2/1 -> If Action Subsystem/1(In1), If/1
  Maximum Allowable/1 -> If Action Subsystem1/1(In1)
  If/1 -> If Action Subsystem1/Action

== system Aim_23__Monocopter_Testing/Cyclic Roll Control/PD Pitch Controller (Monoco negative direction counter clockwise) Front Motor/Offset ==
  In2 : Inport
  Offset : Constant  Value=0.2
  Subtract1 : Sum
  Out1 : Outport
  wires:
  In2/1 -> Subtract1/1
  Offset/1 -> Subtract1/2
  Subtract1/1 -> Out1/1

== system Aim_23__Monocopter_Testing/Cyclic Roll Control/PD Pitch Controller (Monoco negative direction counter clockwise)2/Low Pass Filter ==
  In2 : Inport
  If : If  IfExpression=u1<(-2300)
  If Action Subsystem : Subsystem  TreatAsAtomicUnit=on
  If Action Subsystem1 : Subsystem  TreatAsAtomicUnit=on
  Maximum Allowable : Constant  Value=-2300
  Merge : Merge
  u : Outport
  wires:
  Merge/1 -> u/1
  If/2 -> If Action Subsystem/Action
  If Action Subsystem/1(Out1) -> Merge/2
  If Action Subsystem1/1(Out1) -> Merge/1
  In2/1 -> If Action Subsystem/1(In1), If/1
  Maximum Allowable/1 -> If Action Subsystem1/1(In1)
  If/1 -> If Action Subsystem1/Action

== system Aim_23__Monocopter_Testing/Cyclic Roll Control/PD Pitch Controller (Monoco negative direction counter clockwise)2/Offset ==
  In2 : Inport
  Offset : Constant  Value=0.2
  Subtract1 : Sum
  Out1 : Outport
  wires:
  In2/1 -> Subtract1/1
  Offset/1 -> Subtract1/2
  Subtract1/1 -> Out1/1

== system Aim_23__Monocopter_Testing/Cyclic Roll Control/PD Pitch Controller (Monoco positve direction clockwise)/Offset ==
  In2 : Inport
  Offset : Constant  Value=0.2
  Subtract1 : Sum
  Out1 : Outport
  wires:
  In2/1 -> Subtract1/1
  Offset/1 -> Subtract1/2
  Subtract1/1 -> Out1/1

== system Aim_23__Monocopter_Testing/Cyclic Roll Control/PD Roll Controller (Monoco negative direction counter clockwise) Back Motor/Low Pass Filter ==
  In2 : Inport
  If : If  IfExpression=u1<(-2300)
  If Action Subsystem : Subsystem  TreatAsAtomicUnit=on
  If Action Subsystem1 : Subsystem  TreatAsAtomicUnit=on
  Maximum Allowable : Constant  Value=-2300
  Merge : Merge
  u : Outport
  wires:
  Merge/1 -> u/1
  If/2 -> If Action Subsystem/Action
  If Action Subsystem/1(Out1) -> Merge/2
  If Action Subsystem1/1(Out1) -> Merge/1
  In2/1 -> If Action Subsystem/1(In1), If/1
  Maximum Allowable/1 -> If Action Subsystem1/1(In1)
  If/1 -> If Action Subsystem1/Action

== system Aim_23__Monocopter_Testing/Cyclic Roll Control/PD Roll Controller (Monoco negative direction counter clockwise) Front Motor/Low Pass Filter ==
  In2 : Inport
  If : If  IfExpression=u1<(-2300)
  If Action Subsystem : Subsystem  TreatAsAtomicUnit=on
  If Action Subsystem1 : Subsystem  TreatAsAtomicUnit=on
  Maximum Allowable : Constant  Value=-2300
  Merge : Merge
  u : Outport
  wires:
  Merge/1 -> u/1
  If/2 -> If Action Subsystem/Action
  If Action Subsystem/1(Out1) -> Merge/2
  If Action Subsystem1/1(Out1) -> Merge/1
  In2/1 -> If Action Subsystem/1(In1), If/1
  Maximum Allowable/1 -> If Action Subsystem1/1(In1)
  If/1 -> If Action Subsystem1/Action

== system Aim_23__Monocopter_Testing/Cyclic Roll Control/PD Roll Controller (Monoco positve direction clockwise)/Offset ==
  In2 : Inport
  Offset : Constant  Value=0.2
  Subtract1 : Sum
  Out1 : Outport
  wires:
  In2/1 -> Subtract1/1
  Offset/1 -> Subtract1/2
  Subtract1/1 -> Out1/1
